simulink model "CK_index_bass"  (R2023a)
settings: Solver=VariableStepAuto  StartTime=0.0  StopTime=500  RelTol=1e-3
values from neighbouring files (symbols this model uses):
  a0 = 0.01    [script.m]
  a1 = 5    [script.m]
  a2 = 10    [script.m]
  a_i_Top = 1    [script.m]
  Alpha = 2    [script.m]
  Alpha1 = 10    [script.m]
  Alpha2 = 5    [script.m]
  Alpha3 = 1    [script.m]
  b0 = 0.001    [script.m]
  b1 = 0.25    [script.m]
  b2 = 1    [script.m]
  Cr = 1    [script.m]
  d1 = 0.1    [script.m]
  d2 = 1    [script.m]
  ds = 0.1    [script.m]
  dw = 0.33    [script.m]
  K1 = 1    [script.m]
  K2 = 1    [script.m]
  Kh1 = 5    [script.m]
  Kh2 = 5    [script.m]
  n = 2    [script.m]
  ra = 0.025    [script.m]
  rclv = 0.025    [script.m]
  rclvs = 0.025    [script.m]
  rcyt = 0.025    [script.m]
  receptor_i1 = 0.5    [script.m]
  rsc = 0.025    [script.m]
  rw = 0.025    [script.m]
  V1 = 1    [script.m]
  Vh1 = 2    [script.m]
settings Model: Creator=mosuk  LastModifiedBy=mosuk

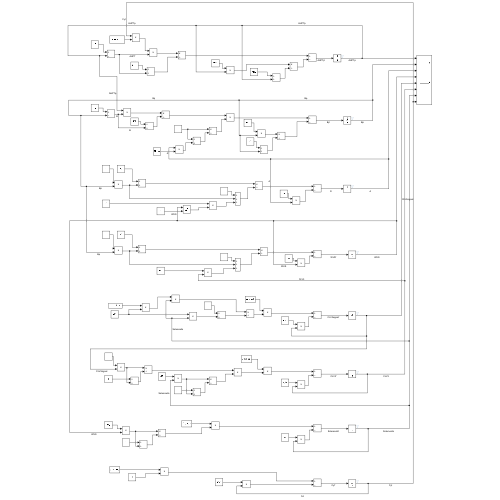
[thumbnail: Simulink's stored preview of the top-level diagram]
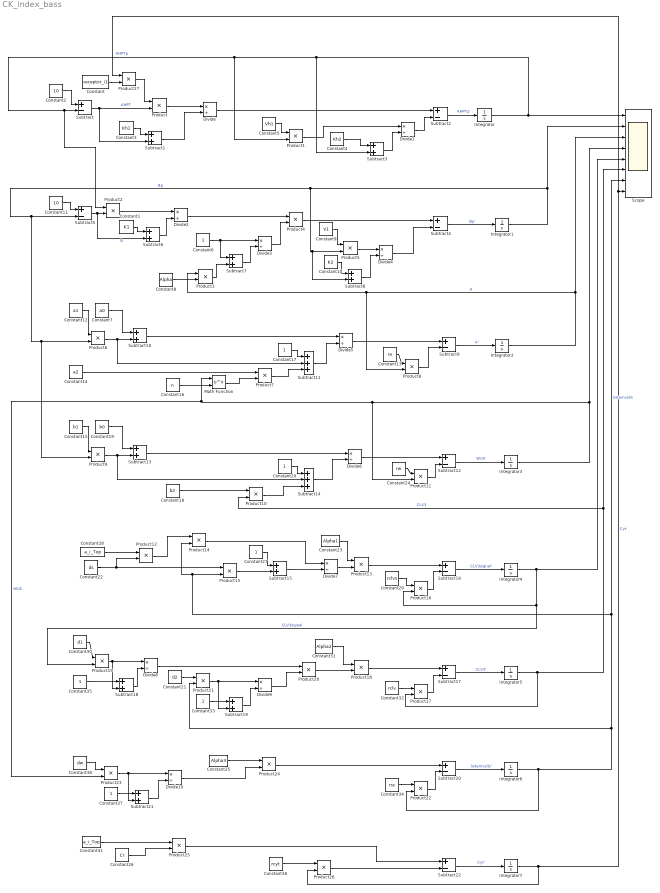
== system CK_index_bass ==
  Constant : Constant  Value=receptor_i1
  Constant1 : Constant  Value=K1
  Constant10 : Constant  Value=K2
  Constant11 : Constant  Value=10
  Constant12 : Constant  Value=a1
  Constant13 : Constant  Value=ra
  Constant14 : Constant  Value=a2
  Constant15 : Constant  Value=b1
  Constant16 : Constant  Value=n
  Constant{6,17,20,27,33,35,37} (7 alike) : Constant
  Constant18 : Constant  Value=b2
  Constant19 : Constant  Value=b0
  Constant2 : Constant  Value=10
  Constant21 : Constant  Value=d2
  Constant22 : Constant  Value=ds
  Constant23 : Constant  Value=Alpha1
  Constant24 : Constant  Value=rw
  Constant25 : Constant  Value=Alpha3
  Constant26 : Constant  Value=Cr
  Constant28 : Constant  Value=a_i_Top
  Constant29 : Constant  Value=rclvs
  Constant3 : Constant  Value=Kh1
  Constant30 : Constant  Value=d1
  Constant31 : Constant  Value=Alpha2
  Constant32 : Constant  Value=rclv
  Constant34 : Constant  Value=rsc
  Constant36 : Constant  Value=rcyt
  Constant38 : Constant  Value=dw
  Constant4 : Constant  Value=Kh2
  Constant41 : Constant  Value=a_i_Top
  Constant5 : Constant  Value=Vh1
  Constant7 : Constant  Value=a0
  Constant8 : Constant  Value=Alpha
  Constant9 : Constant  Value=V1
  Divide{,1..10} (11 alike) : Product  Inputs=*/
  Integrator{,1..7} (8 alike) : Integrator
  Math Function : Math  Operator=pow
  Product{,1..27} (28 alike) : Product
  Scope : Scope  NumInputPorts=8
  Subtract{,2,4..5,9,12,16..17,20,22} (10 alike) : Sum  Inputs=+-
  Subtract{1,3,6..8,10,13,15,18..19,21} (11 alike) : Sum
  Subtract11 : Sum  Inputs=+++
  Subtract14 : Sum  Inputs=+++
  wires:
  Product27/1 -> Product/1
  Integrator/1 -> Subtract3/2, Product1/2, Product2/1, Subtract/2, Scope/1  "AHPTp"
  Subtract2/1 -> Integrator/1  "AHPTp'"
  Constant2/1 -> Subtract/1
  Subtract/1 -> Subtract1/2, Product/2  "AHPT"
  Product/1 -> Divide/1
  Constant3/1 -> Subtract1/1
  Subtract1/1 -> Divide/2
  Divide/1 -> Subtract2/1
  Constant5/1 -> Product1/1
  Constant4/1 -> Subtract3/1
  Subtract3/1 -> Divide1/2
  Product1/1 -> Divide1/1
  Divide1/1 -> Subtract2/2
  Integrator1/1 -> Scope/2, Subtract8/2, Product5/2, Subtract5/2, Product9/2, Product6/2  "Bp"
  Subtract4/1 -> Integrator1/1  "Bp'"
  Constant11/1 -> Subtract5/1
  Subtract5/1 -> Subtract6/2, Product2/2  "B"
  Constant1/1 -> Subtract6/1
  Product2/1 -> Divide2/1
  Subtract6/1 -> Divide2/2
  Constant8/1 -> Product3/2
  Integrator2/1 -> Product8/2, Product3/1, Scope/3  "A"
  Constant6/1 -> Subtract7/1, Divide3/1
  Product3/1 -> Subtract7/2
  Subtract7/1 -> Divide3/2
  Divide2/1 -> Product4/1
  Divide3/1 -> Product4/2
  Product4/1 -> Subtract4/1
  Constant9/1 -> Product5/1
  Constant10/1 -> Subtract8/1
  Product5/1 -> Divide4/1
  Subtract8/1 -> Divide4/2
  Divide4/1 -> Subtract4/2
  Subtract9/1 -> Integrator2/1  "A'"
  Constant12/1 -> Product6/1
  Constant7/1 -> Subtract10/1
  Product6/1 -> Subtract11/2, Subtract10/2
  Subtract10/1 -> Divide5/1
  Constant17/1 -> Subtract11/1
  Integrator3/1 -> Product11/2, Product23/2, Math Function/1, Scope/4  "WUS"
  Constant16/1 -> Math Function/2
  Product7/1 -> Subtract11/3
  Constant14/1 -> Product7/1
  Math Function/1 -> Product7/2
  Subtract11/1 -> Divide5/2
  Divide5/1 -> Subtract9/1
  Constant13/1 -> Product8/1
  Product8/1 -> Subtract9/2
  Subtract12/1 -> Integrator3/1  "WUS'"
  Constant15/1 -> Product9/1
  Constant19/1 -> Subtract13/1
  Product9/1 -> Subtract14/2, Subtract13/2
  Subtract13/1 -> Divide6/1
  Divide6/1 -> Subtract12/1
  Constant20/1 -> Subtract14/1
  Constant18/1 -> Product10/1
  Product10/1 -> Subtract14/3
  Integrator4/1 -> Product19/2, Product16/2, Scope/5  "CLV3signal"
  Subtract14/1 -> Divide6/2
  Product11/1 -> Subtract12/2
  Constant24/1 -> Product11/1
  Constant23/1 -> Product13/1
  Subtract16/1 -> Integrator4/1  "CLV3signal'"
  Constant28/1 -> Product12/1
  Constant22/1 -> Product12/2, Product15/1
  Product12/1 -> Product14/1
  Constant27/1 -> Subtract15/1
  Product15/1 -> Subtract15/2
  Subtract15/1 -> Divide7/2
  Product13/1 -> Subtract16/1
  Divide7/1 -> Product13/2
  Product14/1 -> Divide7/1
  Constant29/1 -> Product16/1
  Product16/1 -> Subtract16/2
  Subtract17/1 -> Integrator5/1  "CLV3'"
  Integrator5/1 -> Product10/2, Scope/6, Product17/2  "CLV3"
  Constant32/1 -> Product17/1
  Product17/1 -> Subtract17/2
  Product18/1 -> Subtract17/1
  Constant31/1 -> Product18/1
  Constant30/1 -> Product19/1
  Product19/1 -> Divide8/1, Subtract18/2
  Constant35/1 -> Subtract18/1
  Subtract18/1 -> Divide8/2
  Product20/1 -> Product18/2
  Divide8/1 -> Product20/1
  Constant21/1 -> Product21/1
  Integrator6/1 -> Product22/2, Product21/2, Product15/2, Product14/2, Scope/7  "Sstemcells"
  Product21/1 -> Subtract19/2, Divide9/1
  Constant33/1 -> Subtract19/1
  Subtract19/1 -> Divide9/2
  Divide9/1 -> Product20/2
  Subtract20/1 -> Integrator6/1  "Sstemcells'"
  Constant34/1 -> Product22/1
  Product22/1 -> Subtract20/2
  Constant38/1 -> Product23/1
  Constant37/1 -> Subtract21/1
  Product23/1 -> Subtract21/2, Divide10/1
  Subtract21/1 -> Divide10/2
  Constant25/1 -> Product24/1
  Divide10/1 -> Product24/2
  Product24/1 -> Subtract20/1
  Constant41/1 -> Product25/1
  Constant26/1 -> Product25/2
  Integrator7/1 -> Product26/2, Product27/1, Scope/8  "Cyt"
  Subtract22/1 -> Integrator7/1  "Cyt'"
  Constant36/1 -> Product26/1
  Product26/1 -> Subtract22/2
  Product25/1 -> Subtract22/1
  Constant/1 -> Product27/2
